simulink model "Input_Shaping"  (R2018a)
settings: Solver=ode4  StartTime=0.0  StopTime=20  FixedStep=0.002  RelTol=1e-3  EnableMultiTasking=on
values from neighbouring files (symbols this model uses):
  A0 = 1/(1+2*K+K^2)    [InputShaper.m]
  A1 = 2*K/(1+2*K+K^2)    [InputShaper.m]
  A2 = K^2/(1+2*K+K^2)    [InputShaper.m]
  t1 = Td/2    (= 0.23)    [InputShaper.m]
  t2 = Td    (= 0.46)    [InputShaper.m]
undefined symbols (not defined in the file or in its folder): HIL, qc_get_step_size
libraries: quarc_library x12, dspsrcs4 x1, simulink x1
settings Model: SimulationMode=external  ExtModeTrigDuration=20000  Creator=MLevis  LastModifiedBy=Student
settings SolverCC: PositivePriorityOrder=on  AutoInsertRateTranBlk=on
settings DataIOCC: LimitDataPoints=on  SaveFormat=Array
settings OptimizationCC: LifeSpan=inf
settings DebuggingCC: SolverPrmCheckMsg=warning  SFUnexpectedBacktrackingDiag=warning  SFNoUnconditionalDefaultTransitionDiag=warning  SFExecutionAtInitializationDiag=none
settings HardwareCC: ProdBitPerPointer=32  ProdBitPerSizeT=32  ProdBitPerPtrDiffT=32  ProdLargestAtomicFloat=None  ProdIntDivRoundTo=Undefined  ProdEndianess=Unspecified  ProdWordSize=32  ProdHWDeviceType=32-bit Generic
settings ModelReferenceCC: PropagateSignalLabelsOutOfModel=off
settings RTWCC: SystemTargetFile=quarc_win64.tlc  TemplateMakefile=quarc_default_tmf  Description=QUARC Win64 Target
settings CodeAppCC: StateflowObjectComments=on
settings STFCustomTargetCC: TargetPreCompLibLocation=C:\PROGRA~3\QUARC\lib\2018a\win64\release  ConcurrentExecutionCompliant=on  GeneratePreprocessorConditionals=Disable all  SystemTargetFile=quarc_win64.tlc
settings GRTTargetCC: TargetPreCompLibLocation=C:\PROGRA~3\QUARC\lib\2018a\win64\release  TargetLangStandard=C89/C90 (ANSI)  ParMdlRefBuildCompliant=off  CompOptLevelCompliant=off  GeneratePreprocessorConditionals=Disable all  CombineOutputUpdateFcns=off  MatFileLogging=off  CPPClassGenCompliant=off  GRTInterface=on  UseToolchainInfoCompliant=off  ExtMode=on  ExtModeMexFile=quarc_comm
settings ConfigComp: CovMetricSettings=dw  CovHtmlReporting=on  CovSaveCumulativeToWorkspaceVar=on  CovSaveSingleToWorkspaceVar=on  CovExternalEMLEnable=off  CovSFcnEnable=off

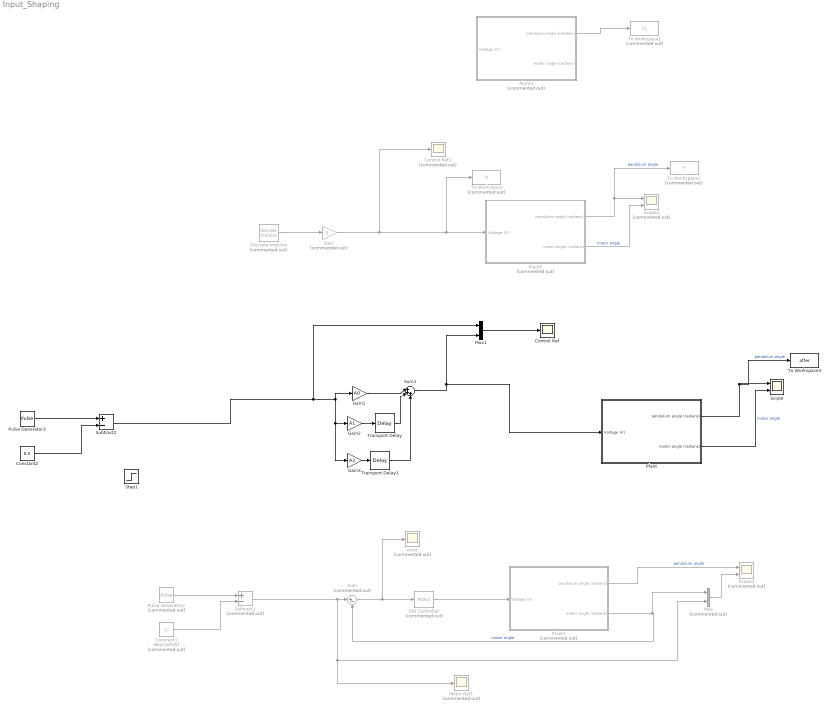
== system Input_Shaping ==
  Constant1 : Constant  Commented=on  Value=deg2rad(45)
  Constant2 : Constant  Value=0.5
  Control Ref : Scope
  Control Ref1 : Scope  Commented=on
  Discrete Impulse : dspsrcs4/Discrete  Impulse  Commented=on  Delay=1  SampleTime=0.1  FrameSample=1  OutputFrames=off  dataType=double  isSigned=on  wordLen=16  udDataType=sfix(16)  fracBitsMode=Best precision  numFracBits=15  OutDataTypeStr=double  LastOutDataTypeStr=double
  Gain : Gain  Commented=on  Gain=5
  Gain1 : Gain  Gain=A0
  Gain2 : Gain  Gain=A1
  Gain3 : Gain  Gain=A2
  Motor Ref1 : Scope  Commented=on
  Mux : Mux  Commented=on  Inputs=2
  Mux1 : Mux  Inputs=2
  PID Controller : simulink/Continuous/PID Controller  Commented=on  Controller=PID  TimeDomain=Continuous-time  SampleTime=-1  IntegratorMethod=Forward Euler  FilterMethod=Forward Euler  Form=Parallel  UseFilter=on  ControllerParametersSource=internal  P=1  I=1.2  D=0.2  N=100  InitialConditionSource=internal  InitialConditionForIntegrator=0  InitialConditionForFilter=0  ExternalReset=none  LimitOutput=off  UpperSaturationLimit=inf  LowerSaturationLimit=-inf  LinearizeAsGain=on  AntiWindupMode=none  Kb=1  TrackingMode=off  Kt=1  PParamMin=[]  PParamMax=[]  IParamMin=[]  IParamMax=[]  DParamMin=[]  DParamMax=[]  NParamMin=[]  NParamMax=[]  KbParamMin=[]  KbParamMax=[]  KtParamMin=[]  KtParamMax=[]  POutMin=[]  POutMax=[]  IOutMin=[]  IOutMax=[]  DOutMin=[]  DOutMax=[]  NOutMin=[]  NOutMax=[]  KbOutMin=[]  KbOutMax=[]  KtOutMin=[]  KtOutMax=[]  IntegratorOutMin=[]  IntegratorOutMax=[]  FilterOutMin=[]  FilterOutMax=[]  SumOutMin=[]  SumOutMax=[]  SumI1OutMin=[]  SumI1OutMax=[]  SumI2OutMin=[]  SumI2OutMax=[]  SumI3OutMin=[]  SumI3OutMax=[]  SumDOutMin=[]  SumDOutMax=[]  SaturationOutMin=[]  SaturationOutMax=[]  IntegratorContinuousStateAttributes=''  IntegratorStateMustResolveToSignalObject=off  IntegratorRTWStateStorageClass=Auto  FilterContinuousStateAttributes=''  FilterStateMustResolveToSignalObject=off  FilterRTWStateStorageClass=Auto  DifferentiatorICPrevScaledInput=0  DifferentiatorOutMin=[]  DifferentiatorOutMax=[]  FilterDiffOutCoefMin=[]  FilterDiffOutCoefMax=[]  SumDenOutMin=[]  SumDenOutMax=[]  SumNumOutMin=[]  SumNumOutMax=[]  ReciprocalOutMin=[]  ReciprocalOutMax=[]  DivideOutMin=[]  DivideOutMax=[]  TunerSelectOption=Transfer Function Based (PID Tuner App)
  Plant : Subsystem
  Plant1 : Subsystem  Commented=on
  Plant2 : Subsystem  Commented=on
  Plant3 : Subsystem  Commented=on
  Pulse Generator2 : DiscretePulseGenerator  Commented=on  PulseType=Time based  Amplitude=2 * deg2rad(45)  Period=10  PulseWidth=50
  Pulse Generator3 : DiscretePulseGenerator  PulseType=Time based  Period=5  PulseWidth=50
  Scope : Scope  NumInputPorts=2
  Scope1 : Scope  Commented=on  NumInputPorts=2
  Scope2 : Scope  Commented=on  NumInputPorts=2
  Step1 : Step  After=0.8  SampleTime=0
  Subtract1 : Sum  Commented=on  Inputs=+-
  Subtract2 : Sum  Inputs=+-
  Sum : Sum  Commented=on  Inputs=|+-
  Sum1 : Sum  Inputs=|+++
  To Workspace : ToWorkspace  Commented=on  VariableName=U  SampleTime=0.002
      settings: Save2DSignal=2-D array (concatenate along first dimension)
  To Workspace1 : ToWorkspace  Commented=on  VariableName=Y  SampleTime=0.002
      settings: Save2DSignal=2-D array (concatenate along first dimension)
  To Workspace2 : ToWorkspace  Commented=on  VariableName=Y1  SampleTime=0.002
      settings: Save2DSignal=2-D array (concatenate along first dimension)
  To Workspace3 : ToWorkspace  VariableName=after  SampleTime=-1
  Transport Delay : TransportDelay  DelayTime=t1
  Transport Delay1 : TransportDelay  DelayTime=t2
  error : Scope  Commented=on
  wires:
  Plant/1(pendulum angle (radians)) -> To Workspace3/1, Scope/1  "pendulum angle"
  Plant/2(motor angle (radians)) -> Scope/2  "motor angle"
  Subtract1/1 -> Sum/1, Mux/2, Motor Ref1/1
  Pulse Generator2/1 -> Subtract1/1
  Constant1/1 -> Subtract1/2
  Plant1/2(motor angle (radians)) -> Mux/1, Sum/2  "motor angle"
  Plant1/1(pendulum angle (radians)) -> Scope1/1  "pendulum angle"
  Sum/1 -> error/1, PID Controller/1
  PID Controller/1 -> Plant1/1(Voltage (V))
  Mux/1 -> Scope1/2
  Plant2/2(motor angle (radians)) -> Scope2/2  "motor angle"
  Plant2/1(pendulum angle (radians)) -> To Workspace1/1, Scope2/1  "pendulum angle"
  Discrete Impulse/1 -> Gain/1
  Gain/1 -> Control Ref1/1, To Workspace/1, Plant2/1(Voltage (V))
  Gain3/1 -> Transport Delay1/1
  Gain2/1 -> Transport Delay/1
  Subtract2/1 -> Mux1/1, Gain1/1, Gain2/1, Gain3/1
  Transport Delay1/1 -> Sum1/3
  Transport Delay/1 -> Sum1/2
  Gain1/1 -> Sum1/1
  Sum1/1 -> Plant/1(Voltage (V)), Mux1/2
  Mux1/1 -> Control Ref/1
  Constant2/1 -> Subtract2/2
  Pulse Generator3/1 -> Subtract2/1
  Plant3/1(pendulum angle (radians)) -> To Workspace2/1

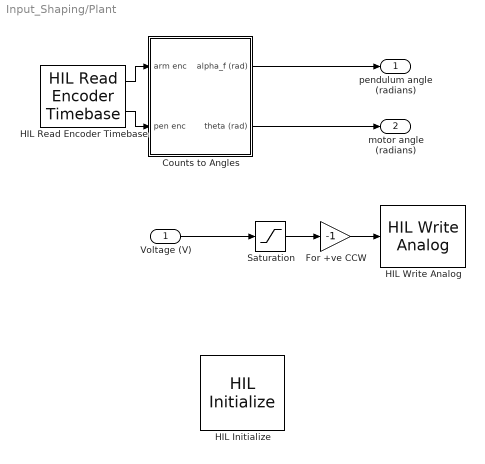
== system Input_Shaping/Plant ==
  Voltage (V) : Inport
  Counts to Angles : Subsystem
  For +ve CCW : Gain  Gain=-1
  HIL Initialize : quarc_library/Data Acquisition/Generic/Configuration/HIL Initialize  object_name=HIL-1  board_type=qube_servo2_usb  board_number=0  board_options=""  exclusive=off  active=off  hardware_clocks=[0]  clock_modes=[]  initial_clock_frequencies=[]  set_clock_params_at_start=off  set_clock_params_at_switch_in=off  set_clock_frequencies_at_start=off  set_clock_frequencies_at_switch_in=off  analog_input_channels=[0]  analog_input_configurations=[]  analog_input_maximums=3  analog_input_minimums=-3  set_analog_input_params_at_start=off  set_analog_input_params_at_switch_in=off  analog_output_channels=[0]  analog_output_maximums=15  analog_output_minimums=-15  initial_analog_outputs=[0]  final_analog_outputs=[0]  watchdog_analog_outputs=0  set_analog_output_params_at_start=off  set_analog_output_params_at_switch_in=off  set_analog_outputs_at_start=on  set_analog_outputs_at_switch_in=off  set_analog_outputs_at_terminate=on  set_analog_outputs_at_switch_out=off  set_analog_outputs_on_watchdog=on  digital_input_channels=[]  digital_output_channels=[0]  digital_output_configuration=[]  initial_digital_outputs=[1]  final_digital_outputs=[0]  watchdog_digital_outputs=[0]  set_digital_output_params_at_start=off  set_digital_output_params_at_switch_in=off  set_digital_outputs_at_start=on  set_digital_outputs_at_switch_in=off  set_digital_outputs_at_terminate=on  set_digital_outputs_at_switch_out=off  set_digital_outputs_on_watchdog=on  encoder_channels=[0:1]  quadrature=[4]  encoder_filter_frequency=[]  initial_encoder_counts=[0]  set_encoder_params_at_start=off  set_encoder_params_at_switch_in=off  set_encoder_counts_at_start=on  set_encoder_counts_at_switch_in=off  pwm_channels=[]  pwm_modes=[]  pwm_frequency=[]  pwm_configuration=[]  pwm_alignment=[]  pwm_polarity=[]  pwm_leading_deadband=[]  pwm_trailing_deadband=[]  initial_pwm_outputs=[]  final_pwm_outputs=[]  watchdog_pwm_outputs=[]  set_pwm_params_at_start=off  set_pwm_params_at_switch_in=off  set_pwm_outputs_at_start=off  set_pwm_outputs_at_switch_in=off  set_pwm_outputs_at_terminate=off  set_pwm_outputs_at_switch_out=off  set_pwm_outputs_on_watchdog=off  other_output_channels=[11000:11002]  initial_other_outputs=[0 1 0]  final_other_outputs=[1 0 0]  watchdog_other_outputs=[0 0 1]  set_other_outputs_at_start=on  set_other_outputs_at_switch_in=off  set_other_outputs_at_terminate=on  set_other_outputs_at_switch_out=off  set_other_outputs_on_watchdog=on
  HIL Read Encoder Timebase : quarc_library/Data Acquisition/Generic/Timebases/HIL Read Encoder Timebase  object_name=HIL-1  clock=0  channels=[0:1]  samples_in_buffer=max(ceil(1/qc_get_step_size), 1)  active=on  vector_output=off  data_type_mode=Inherit via back propagation  data_type=double
  HIL Write Analog : quarc_library/Data Acquisition/Generic/Immediate I//O/HIL Write Analog  object_name=HIL-1  channels=0  sample_time=-1  active=off  vector_input=off
  Saturation : Saturate  UpperLimit=10  LowerLimit=-10
  pendulum angle (radians) : Outport
  motor angle (radians) : Outport  Port=2
  wires:
  Counts to Angles/2(theta (rad)) -> motor angle (radians)/1
  Counts to Angles/1(alpha_f (rad)) -> pendulum angle (radians)/1
  HIL Read Encoder Timebase/2 -> Counts to Angles/2(pen enc)
  HIL Read Encoder Timebase/1 -> Counts to Angles/1(arm enc)
  Voltage (V)/1 -> Saturation/1
  Saturation/1 -> For +ve CCW/1
  For +ve CCW/1 -> HIL Write Analog/1

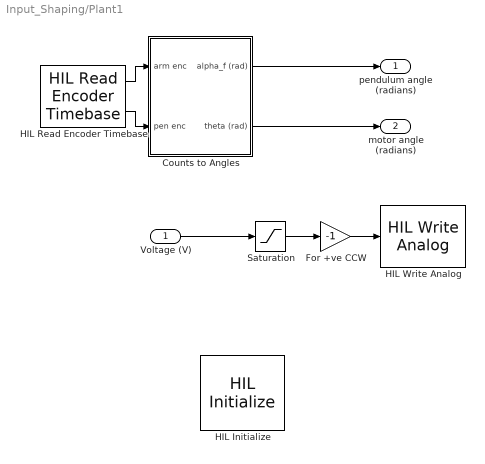
== system Input_Shaping/Plant1 ==
  Voltage (V) : Inport
  Counts to Angles : Subsystem
  For +ve CCW : Gain  Gain=-1
  HIL Initialize : quarc_library/Data Acquisition/Generic/Configuration/HIL Initialize  object_name=HIL-2  board_type=qube_servo2_usb  board_number=0  board_options=""  exclusive=off  active=off  hardware_clocks=[0]  clock_modes=[]  initial_clock_frequencies=[]  set_clock_params_at_start=off  set_clock_params_at_switch_in=off  set_clock_frequencies_at_start=off  set_clock_frequencies_at_switch_in=off  analog_input_channels=[0]  analog_input_configurations=[]  analog_input_maximums=3  analog_input_minimums=-3  set_analog_input_params_at_start=off  set_analog_input_params_at_switch_in=off  analog_output_channels=[0]  analog_output_maximums=15  analog_output_minimums=-15  initial_analog_outputs=[0]  final_analog_outputs=[0]  watchdog_analog_outputs=0  set_analog_output_params_at_start=off  set_analog_output_params_at_switch_in=off  set_analog_outputs_at_start=on  set_analog_outputs_at_switch_in=off  set_analog_outputs_at_terminate=on  set_analog_outputs_at_switch_out=off  set_analog_outputs_on_watchdog=on  digital_input_channels=[]  digital_output_channels=[0]  digital_output_configuration=[]  initial_digital_outputs=[1]  final_digital_outputs=[0]  watchdog_digital_outputs=[0]  set_digital_output_params_at_start=off  set_digital_output_params_at_switch_in=off  set_digital_outputs_at_start=on  set_digital_outputs_at_switch_in=off  set_digital_outputs_at_terminate=on  set_digital_outputs_at_switch_out=off  set_digital_outputs_on_watchdog=on  encoder_channels=[0:1]  quadrature=[4]  encoder_filter_frequency=[]  initial_encoder_counts=[0]  set_encoder_params_at_start=off  set_encoder_params_at_switch_in=off  set_encoder_counts_at_start=on  set_encoder_counts_at_switch_in=off  pwm_channels=[]  pwm_modes=[]  pwm_frequency=[]  pwm_configuration=[]  pwm_alignment=[]  pwm_polarity=[]  pwm_leading_deadband=[]  pwm_trailing_deadband=[]  initial_pwm_outputs=[]  final_pwm_outputs=[]  watchdog_pwm_outputs=[]  set_pwm_params_at_start=off  set_pwm_params_at_switch_in=off  set_pwm_outputs_at_start=off  set_pwm_outputs_at_switch_in=off  set_pwm_outputs_at_terminate=off  set_pwm_outputs_at_switch_out=off  set_pwm_outputs_on_watchdog=off  other_output_channels=[11000:11002]  initial_other_outputs=[0 1 0]  final_other_outputs=[1 0 0]  watchdog_other_outputs=[0 0 1]  set_other_outputs_at_start=on  set_other_outputs_at_switch_in=off  set_other_outputs_at_terminate=on  set_other_outputs_at_switch_out=off  set_other_outputs_on_watchdog=on
  HIL Read Encoder Timebase : quarc_library/Data Acquisition/Generic/Timebases/HIL Read Encoder Timebase  object_name=HIL-2  clock=0  channels=[0:1]  samples_in_buffer=max(ceil(1/qc_get_step_size), 1)  active=on  vector_output=off  data_type_mode=Inherit via back propagation  data_type=double
  HIL Write Analog : quarc_library/Data Acquisition/Generic/Immediate I//O/HIL Write Analog  object_name=HIL-2  channels=0  sample_time=-1  active=off  vector_input=off
  Saturation : Saturate  UpperLimit=10  LowerLimit=-10
  pendulum angle (radians) : Outport
  motor angle (radians) : Outport  Port=2
  wires:
  Counts to Angles/2(theta (rad)) -> motor angle (radians)/1
  Counts to Angles/1(alpha_f (rad)) -> pendulum angle (radians)/1
  HIL Read Encoder Timebase/2 -> Counts to Angles/2(pen enc)
  HIL Read Encoder Timebase/1 -> Counts to Angles/1(arm enc)
  Voltage (V)/1 -> Saturation/1
  Saturation/1 -> For +ve CCW/1
  For +ve CCW/1 -> HIL Write Analog/1

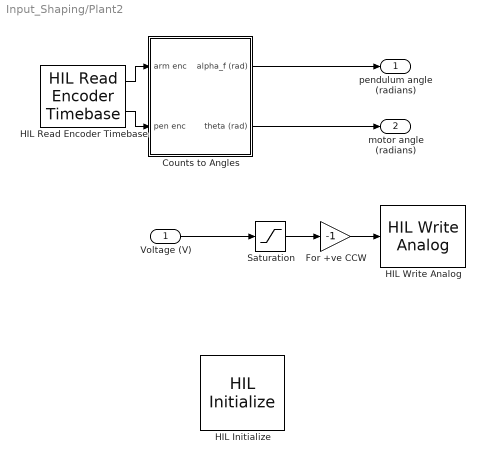
== system Input_Shaping/Plant2 ==
  Voltage (V) : Inport
  Counts to Angles : Subsystem
  For +ve CCW : Gain  Gain=-1
  HIL Initialize : quarc_library/Data Acquisition/Generic/Configuration/HIL Initialize  object_name=HIL-2  board_type=qube_servo2_usb  board_number=0  board_options=""  exclusive=off  active=off  hardware_clocks=[0]  clock_modes=[]  initial_clock_frequencies=[]  set_clock_params_at_start=off  set_clock_params_at_switch_in=off  set_clock_frequencies_at_start=off  set_clock_frequencies_at_switch_in=off  analog_input_channels=[0]  analog_input_configurations=[]  analog_input_maximums=3  analog_input_minimums=-3  set_analog_input_params_at_start=off  set_analog_input_params_at_switch_in=off  analog_output_channels=[0]  analog_output_maximums=15  analog_output_minimums=-15  initial_analog_outputs=[0]  final_analog_outputs=[0]  watchdog_analog_outputs=0  set_analog_output_params_at_start=off  set_analog_output_params_at_switch_in=off  set_analog_outputs_at_start=on  set_analog_outputs_at_switch_in=off  set_analog_outputs_at_terminate=on  set_analog_outputs_at_switch_out=off  set_analog_outputs_on_watchdog=on  digital_input_channels=[]  digital_output_channels=[0]  digital_output_configuration=[]  initial_digital_outputs=[1]  final_digital_outputs=[0]  watchdog_digital_outputs=[0]  set_digital_output_params_at_start=off  set_digital_output_params_at_switch_in=off  set_digital_outputs_at_start=on  set_digital_outputs_at_switch_in=off  set_digital_outputs_at_terminate=on  set_digital_outputs_at_switch_out=off  set_digital_outputs_on_watchdog=on  encoder_channels=[0:1]  quadrature=[4]  encoder_filter_frequency=[]  initial_encoder_counts=[0]  set_encoder_params_at_start=off  set_encoder_params_at_switch_in=off  set_encoder_counts_at_start=on  set_encoder_counts_at_switch_in=off  pwm_channels=[]  pwm_modes=[]  pwm_frequency=[]  pwm_configuration=[]  pwm_alignment=[]  pwm_polarity=[]  pwm_leading_deadband=[]  pwm_trailing_deadband=[]  initial_pwm_outputs=[]  final_pwm_outputs=[]  watchdog_pwm_outputs=[]  set_pwm_params_at_start=off  set_pwm_params_at_switch_in=off  set_pwm_outputs_at_start=off  set_pwm_outputs_at_switch_in=off  set_pwm_outputs_at_terminate=off  set_pwm_outputs_at_switch_out=off  set_pwm_outputs_on_watchdog=off  other_output_channels=[11000:11002]  initial_other_outputs=[0 1 0]  final_other_outputs=[1 0 0]  watchdog_other_outputs=[0 0 1]  set_other_outputs_at_start=on  set_other_outputs_at_switch_in=off  set_other_outputs_at_terminate=on  set_other_outputs_at_switch_out=off  set_other_outputs_on_watchdog=on
  HIL Read Encoder Timebase : quarc_library/Data Acquisition/Generic/Timebases/HIL Read Encoder Timebase  object_name=HIL-2  clock=0  channels=[0:1]  samples_in_buffer=max(ceil(1/qc_get_step_size), 1)  active=on  vector_output=off  data_type_mode=Inherit via back propagation  data_type=double
  HIL Write Analog : quarc_library/Data Acquisition/Generic/Immediate I//O/HIL Write Analog  object_name=HIL-2  channels=0  sample_time=-1  active=off  vector_input=off
  Saturation : Saturate  UpperLimit=10  LowerLimit=-10
  pendulum angle (radians) : Outport
  motor angle (radians) : Outport  Port=2
  wires:
  Counts to Angles/2(theta (rad)) -> motor angle (radians)/1
  Counts to Angles/1(alpha_f (rad)) -> pendulum angle (radians)/1
  HIL Read Encoder Timebase/2 -> Counts to Angles/2(pen enc)
  HIL Read Encoder Timebase/1 -> Counts to Angles/1(arm enc)
  Voltage (V)/1 -> Saturation/1
  Saturation/1 -> For +ve CCW/1
  For +ve CCW/1 -> HIL Write Analog/1

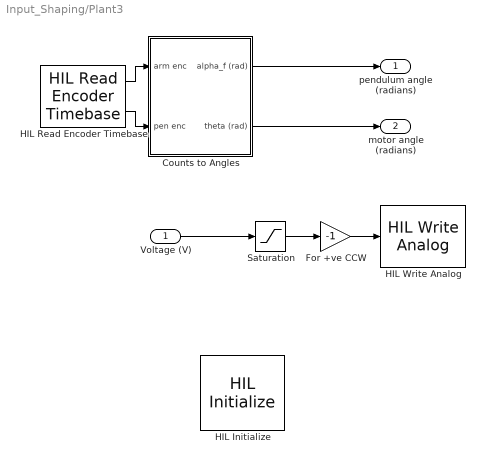
== system Input_Shaping/Plant3 ==
  Voltage (V) : Inport
  Counts to Angles : Subsystem
  For +ve CCW : Gain  Gain=-1
  HIL Initialize : quarc_library/Data Acquisition/Generic/Configuration/HIL Initialize  object_name=HIL-1  board_type=qube_servo2_usb  board_number=0  board_options=""  exclusive=off  active=off  hardware_clocks=[0]  clock_modes=[]  initial_clock_frequencies=[]  set_clock_params_at_start=off  set_clock_params_at_switch_in=off  set_clock_frequencies_at_start=off  set_clock_frequencies_at_switch_in=off  analog_input_channels=[0]  analog_input_configurations=[]  analog_input_maximums=3  analog_input_minimums=-3  set_analog_input_params_at_start=off  set_analog_input_params_at_switch_in=off  analog_output_channels=[0]  analog_output_maximums=15  analog_output_minimums=-15  initial_analog_outputs=[0]  final_analog_outputs=[0]  watchdog_analog_outputs=0  set_analog_output_params_at_start=off  set_analog_output_params_at_switch_in=off  set_analog_outputs_at_start=on  set_analog_outputs_at_switch_in=off  set_analog_outputs_at_terminate=on  set_analog_outputs_at_switch_out=off  set_analog_outputs_on_watchdog=on  digital_input_channels=[]  digital_output_channels=[0]  digital_output_configuration=[]  initial_digital_outputs=[1]  final_digital_outputs=[0]  watchdog_digital_outputs=[0]  set_digital_output_params_at_start=off  set_digital_output_params_at_switch_in=off  set_digital_outputs_at_start=on  set_digital_outputs_at_switch_in=off  set_digital_outputs_at_terminate=on  set_digital_outputs_at_switch_out=off  set_digital_outputs_on_watchdog=on  encoder_channels=[0:1]  quadrature=[4]  encoder_filter_frequency=[]  initial_encoder_counts=[0]  set_encoder_params_at_start=off  set_encoder_params_at_switch_in=off  set_encoder_counts_at_start=on  set_encoder_counts_at_switch_in=off  pwm_channels=[]  pwm_modes=[]  pwm_frequency=[]  pwm_configuration=[]  pwm_alignment=[]  pwm_polarity=[]  pwm_leading_deadband=[]  pwm_trailing_deadband=[]  initial_pwm_outputs=[]  final_pwm_outputs=[]  watchdog_pwm_outputs=[]  set_pwm_params_at_start=off  set_pwm_params_at_switch_in=off  set_pwm_outputs_at_start=off  set_pwm_outputs_at_switch_in=off  set_pwm_outputs_at_terminate=off  set_pwm_outputs_at_switch_out=off  set_pwm_outputs_on_watchdog=off  other_output_channels=[11000:11002]  initial_other_outputs=[0 1 0]  final_other_outputs=[1 0 0]  watchdog_other_outputs=[0 0 1]  set_other_outputs_at_start=on  set_other_outputs_at_switch_in=off  set_other_outputs_at_terminate=on  set_other_outputs_at_switch_out=off  set_other_outputs_on_watchdog=on
  HIL Read Encoder Timebase : quarc_library/Data Acquisition/Generic/Timebases/HIL Read Encoder Timebase  object_name=HIL-1  clock=0  channels=[0:1]  samples_in_buffer=max(ceil(1/qc_get_step_size), 1)  active=on  vector_output=off  data_type_mode=Inherit via back propagation  data_type=double
  HIL Write Analog : quarc_library/Data Acquisition/Generic/Immediate I//O/HIL Write Analog  object_name=HIL-1  channels=0  sample_time=-1  active=off  vector_input=off
  Saturation : Saturate  UpperLimit=10  LowerLimit=-10
  pendulum angle (radians) : Outport
  motor angle (radians) : Outport  Port=2
  wires:
  For +ve CCW/1 -> HIL Write Analog/1
  Saturation/1 -> For +ve CCW/1
  Voltage (V)/1 -> Saturation/1
  HIL Read Encoder Timebase/1 -> Counts to Angles/1(arm enc)
  HIL Read Encoder Timebase/2 -> Counts to Angles/2(pen enc)
  Counts to Angles/1(alpha_f (rad)) -> pendulum angle (radians)/1
  Counts to Angles/2(theta (rad)) -> motor angle (radians)/1

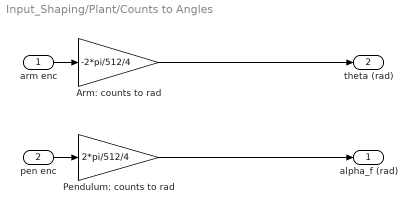
== system Input_Shaping/Plant/Counts to Angles ==
  arm enc : Inport
  pen enc : Inport  Port=2
  Arm: counts to rad : Gain  Gain=-2*pi/512/4
  Pendulum: counts to rad : Gain  Gain=2*pi/512/4
  alpha_f (rad) : Outport
  theta (rad) : Outport  Port=2
  wires:
  pen enc/1 -> Pendulum: counts to rad/1
  arm enc/1 -> Arm: counts to rad/1
  Pendulum: counts to rad/1 -> alpha_f (rad)/1
  Arm: counts to rad/1 -> theta (rad)/1

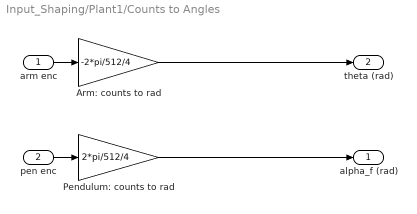
== system Input_Shaping/Plant1/Counts to Angles ==
  arm enc : Inport
  pen enc : Inport  Port=2
  Arm: counts to rad : Gain  Gain=-2*pi/512/4
  Pendulum: counts to rad : Gain  Gain=2*pi/512/4
  alpha_f (rad) : Outport
  theta (rad) : Outport  Port=2
  wires:
  pen enc/1 -> Pendulum: counts to rad/1
  arm enc/1 -> Arm: counts to rad/1
  Pendulum: counts to rad/1 -> alpha_f (rad)/1
  Arm: counts to rad/1 -> theta (rad)/1

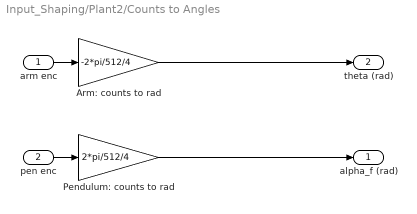
== system Input_Shaping/Plant2/Counts to Angles ==
  arm enc : Inport
  pen enc : Inport  Port=2
  Arm: counts to rad : Gain  Gain=-2*pi/512/4
  Pendulum: counts to rad : Gain  Gain=2*pi/512/4
  alpha_f (rad) : Outport
  theta (rad) : Outport  Port=2
  wires:
  pen enc/1 -> Pendulum: counts to rad/1
  arm enc/1 -> Arm: counts to rad/1
  Pendulum: counts to rad/1 -> alpha_f (rad)/1
  Arm: counts to rad/1 -> theta (rad)/1

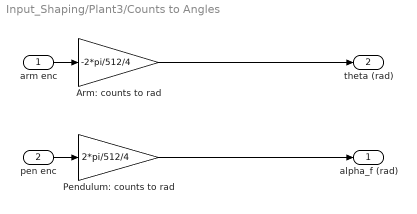
== system Input_Shaping/Plant3/Counts to Angles ==
  arm enc : Inport
  pen enc : Inport  Port=2
  Arm: counts to rad : Gain  Gain=-2*pi/512/4
  Pendulum: counts to rad : Gain  Gain=2*pi/512/4
  alpha_f (rad) : Outport
  theta (rad) : Outport  Port=2
  wires:
  Arm: counts to rad/1 -> theta (rad)/1
  Pendulum: counts to rad/1 -> alpha_f (rad)/1
  arm enc/1 -> Arm: counts to rad/1
  pen enc/1 -> Pendulum: counts to rad/1
